simulink model "GFLIB_ControllerPIr_BAM_FLT"  (Simulink 7.3)
settings: Solver=ode45  StartTime=0.0  StopTime=10.0  RelTol=1e-3
undefined symbols (not defined in the file): fltCC1, fltCC2
settings Model: Creator=RE004C  LastModifiedBy=RE004C
settings HardwareCC: ProdIntDivRoundTo=Zero  ProdEndianess=BigEndian  ProdHWDeviceType=Freescale->32-bit PowerPC

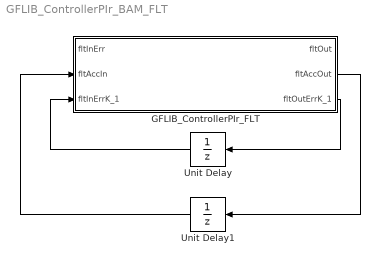
== system GFLIB_ControllerPIr_BAM_FLT ==
  GFLIB_ControllerPIr_FLT : Subsystem  mask(GFLIB_ControllerPIr_FLT){fltCC1=fltCC1, fltCC2=fltCC2}
      mask help: Bit accurate model of reccurent form PI controller. All parameters as well as input and output are single precison floating point numbers.
      mask init:
      | pos = get_param(gcb, 'Position');width = pos(3) - pos(1); height = pos(4) - pos(2);tX=width/2;tY=height*0.9;
      mask Display:
      | color('black');
      | port_label('input',1,'fltInErr');
      | port_label('input',2,'fltAccIn');
      | port_label('input',3,'fltInErrK_1');
      | port_label('output',1,'fltOut');
      | port_label('output',2,'fltAccOut');
      | port_label('output',3,'fltOutErrK_1');
      | color('black');
      | disp('GFLIB_ControllerPIr_FLT');
      | color('blue');
      | text(tX,tY, 'BAM', 'horizontalAlignment', 'center');
  Unit Delay : UnitDelay  SampleTime=-1
  Unit Delay1 : UnitDelay  SampleTime=-1
  wires:
  GFLIB_ControllerPIr_FLT/3(fltOutErrK_1) -> Unit Delay/1
  Unit Delay/1 -> GFLIB_ControllerPIr_FLT/3(fltInErrK_1)
  GFLIB_ControllerPIr_FLT/2(fltAccOut) -> Unit Delay1/1
  Unit Delay1/1 -> GFLIB_ControllerPIr_FLT/2(fltAccIn)

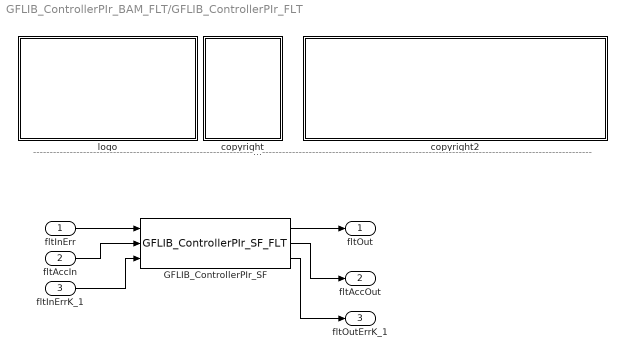
== system GFLIB_ControllerPIr_BAM_FLT/GFLIB_ControllerPIr_FLT ==
  note: ---------------------------------------------------------------------------------------------------------------------------------------------------------------------------------------------------
  fltInErr : Inport  OutDataType=fixdt(1, 16)  OutScaling=2^0
  fltAccIn : Inport  Port=2  OutDataType=fixdt(1, 16)  OutScaling=2^0
  fltInErrK_1 : Inport  Port=3  OutDataType=fixdt(1, 16)  OutScaling=2^0
  GFLIB_ControllerPIr_SF : S-Function  FunctionName=GFLIB_ControllerPIr_SF_FLT  Parameters=fltCC1,fltCC2  EnableBusSupport=off
  copyright : Subsystem
      mask Display: text(10,90,'FILE:');text(10,75,'DESRIPTION:')text(10,60,'COPYRIGHT:')text(10,45,'VERSION:')text(10,30,'DATE:')
  copyright2 : Subsystem
      mask Display: text(10,90,'GFLIB_ControllerPIr_BAM_FLT.mdl');text(10,75,'Recurrent form of a standard PI controller without implemented anti-windup.');text(10,60,'Freescale')text(10,45,'0.1');text(10,30,'20-Jan-2012');
  logo : Subsystem
      mask Display: image(imread('logo.jpg'))
  fltOut : Outport  OutDataType=fixdt(1, 16)  OutScaling=2^0
  fltAccOut : Outport  Port=2  OutDataType=fixdt(1, 16)  OutScaling=2^0
  fltOutErrK_1 : Outport  Port=3  OutDataType=fixdt(1, 16)  OutScaling=2^0
  wires:
  fltInErr/1 -> GFLIB_ControllerPIr_SF/1
  GFLIB_ControllerPIr_SF/1 -> fltOut/1
  fltAccIn/1 -> GFLIB_ControllerPIr_SF/2
  fltInErrK_1/1 -> GFLIB_ControllerPIr_SF/3
  GFLIB_ControllerPIr_SF/2 -> fltAccOut/1
  GFLIB_ControllerPIr_SF/3 -> fltOutErrK_1/1

== system GFLIB_ControllerPIr_BAM_FLT/GFLIB_ControllerPIr_FLT/copyright ==

== system GFLIB_ControllerPIr_BAM_FLT/GFLIB_ControllerPIr_FLT/copyright2 ==

== system GFLIB_ControllerPIr_BAM_FLT/GFLIB_ControllerPIr_FLT/logo ==
